simulink model "Testparentn"  (R2023b)
settings: Solver=FixedStepAuto  StartTime=0.0  StopTime=inf  RelTol=1e-3
undefined symbols (not defined in the file): lat, lon, Testparent2
libraries: androidcommunicationlib x3, androidaudiovideolib x2, androiduilib x2, visionsources x1
settings Model: Creator=Nihar  LastModifiedBy=kaver
settings OptimizationCC: EnhancedBackFolding=on  PassReuseOutputArgsAs=Individual arguments  ZeroExternalMemoryAtStartup=off  ZeroInternalMemoryAtStartup=off  MaxStackSize=64  OptimizeBlockOrder=speed  DifferentSizesBufferReuse=on  OptimizationCustomize=off  EfficientTunableParamExpr=on
settings DebuggingCC: ParameterTunabilityLossMsg=error
settings HardwareCC: ProdBitPerPointer=32  ProdBitPerSizeT=32  ProdBitPerPtrDiffT=32  ProdLargestAtomicInteger=Long  ProdLargestAtomicFloat=Double  ProdWordSize=32  ProdHWDeviceType=ARM Compatible->ARM Cortex
settings SFSimCC: MATLABDynamicMemAlloc=off
settings RTWCC: Description=Embedded Coder  SystemTargetFile=ert.tlc  HardwareBoard=Android Device  TLCOptions="-aInlineSetEventsForThisBaseRateFcn=TLC_FALSE -aSuppressMultiTaskScheduler=TLC_FALSE  -aRateBasedStepFcn=0"  TemplateMakefile=ert_default_tmf  RTWVerbose=off  Toolchain=Android SDK/NDK Tools
settings CodeAppCC: ForceParamTrailComments=on  IgnoreCustomStorageClasses=off  OperatorAnnotations=on  SimulinkDataObjDesc=on  SFDataObjDesc=on  InsertBlockDesc=on

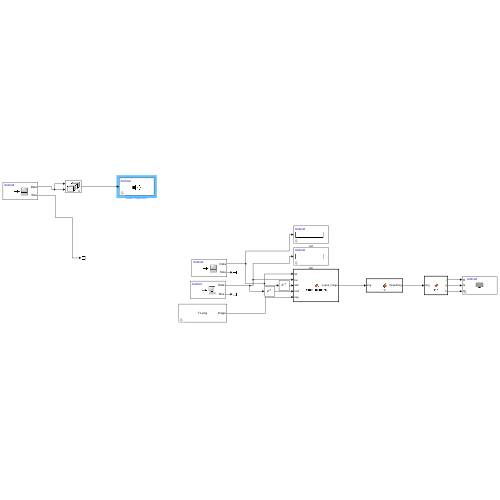
[thumbnail: Simulink's stored preview of the top-level diagram]
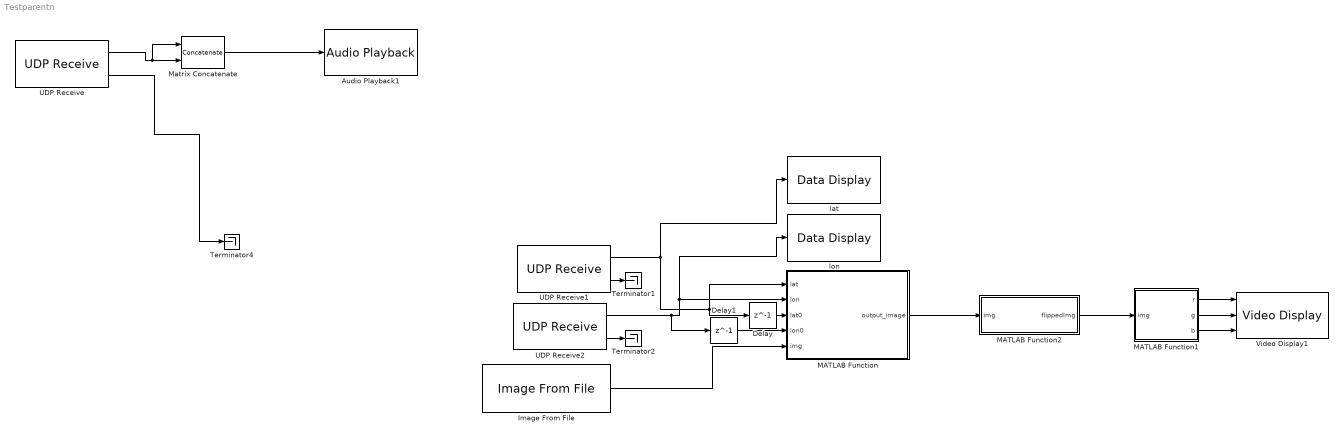
== system Testparentn ==
  Audio Playback1 : androidaudiovideolib/Audio Playback  SampleFreq=44100  AudioSamplingFreq=44100  SampleTime=0.1  DeviceStr=0  QueueDuration=0  BlockPlatform=Android
  Delay : Delay  DelayLength=1
  Delay1 : Delay  DelayLength=1
  Image From File : visionsources/Image From File  Tag=vipblks_nd  FileName=C:\Users\kaver\Downloads\TL.png  Ts=inf  imagePorts=One multidimensional signal  OutPortLabels=R|G|B  ImageDataType=uint8  sdImageDataType=uint(8)  Signed=on  WordLength=16  FractionLengthMode=User-defined  FractionLength=15
  MATLAB Function : MATLAB Function  TreatAsAtomicUnit=on
  MATLAB Function1 : MATLAB Function  TreatAsAtomicUnit=on
  MATLAB Function2 : MATLAB Function  TreatAsAtomicUnit=on
  Matrix Concatenate : Concatenate  Mode=Multidimensional array  ConcatenateDimension=2
  Terminator1 : Terminator
  Terminator2 : Terminator
  Terminator4 : Terminator
  UDP Receive : androidcommunicationlib/UDP Receive  localURL='0.0.0.0'  localPort=20000  remoteURL='0.0.0.0'  remotePort=-1  recvBufferSize=8192  signalDatatype=int16  dims=441  isVarSize=off  showBlockingTime=off  blockingTime=0  sampletime=0.01  blockPlatform=Android
  UDP Receive1 : androidcommunicationlib/UDP Receive  localURL='0.0.0.0'  localPort=35000  remoteURL='0.0.0.0'  remotePort=-1  recvBufferSize=8192  signalDatatype=double  dims=1  isVarSize=off  showBlockingTime=off  blockingTime=0  sampletime=0.01  blockPlatform=Android
  UDP Receive2 : androidcommunicationlib/UDP Receive  localURL='0.0.0.0'  localPort=25000  remoteURL='0.0.0.0'  remotePort=-1  recvBufferSize=8192  signalDatatype=double  dims=1  isVarSize=off  showBlockingTime=off  blockingTime=0  sampletime=0.01  blockPlatform=Android
  Video Display1 : androidaudiovideolib/Video Display  BlockPlatform=Android
  lat : androiduilib/Data Display  DataDisplayId=Testparent2/lat  Format=Float  Precision=6  SimulateUsing=Code generation  blockPlatform=Android
  lon : androiduilib/Data Display  DataDisplayId=Testparent2/lon  Format=Float  Precision=6  SimulateUsing=Code generation  blockPlatform=Android
  wires:
  Matrix Concatenate/1 -> Audio Playback1/1
  MATLAB Function/1(output_image) -> MATLAB Function2/1(img)
  UDP Receive2/2 -> Terminator2/1
  Delay/1 -> MATLAB Function/3(lat0)
  UDP Receive1/2 -> Terminator1/1
  Delay1/1 -> MATLAB Function/4(lon0)
  MATLAB Function1/1(r) -> Video Display1/1
  MATLAB Function1/3(b) -> Video Display1/3
  MATLAB Function1/2(g) -> Video Display1/2
  MATLAB Function2/1(flippedImg) -> MATLAB Function1/1(img)
  UDP Receive2/1 -> Delay1/1, lon/1, MATLAB Function/2(lon)
  Image From File/1 -> MATLAB Function/5(img)
  UDP Receive1/1 -> lat/1, MATLAB Function/1(lat), Delay/1
  UDP Receive/2 -> Terminator4/1
  UDP Receive/1 -> Matrix Concatenate/1, Matrix Concatenate/2

== matlab function Testparentn/MATLAB Function1 ==
  data: img input; r output; g output; b output
function [r,g,b] = fcn(img)
    r = img(:,:,1);
    g = img(:,:,2);
    b = img(:,:,3);
end

== matlab function Testparentn/MATLAB Function ==
  data: lat input; lon input; lat0 input; lon0 input; output_image output; img input
function output_image  = image_mapping(lat,lon,lat0,lon0,img)
    map_width = 883;
    map_height = 675;
    if(lat == 0)
        lat = lat0;
    end
    if(lon == 0)
        lon = lon0;
    end
    X = [83, 620, 640, 80, 441];
    Lx = [23.211144, 23.211170, 23.209616, 23.209530, 23.209997];
    Y = [70, 61, 427, 444, 337];
    Ly = [72.6833273, 72.685835, 72.685929, 72.683318, 72.685008];
    
    yL = zeros(map_height, 1);
    xL = zeros(1,map_width);

    for y = 1:map_height
            w_Y = ((y - Y(2)) * (y - Y(3)) * (y - Y(4)) * (y - Y(5))) / ((Y(1) - Y(2)) * (Y(1) - Y(3)) * (Y(1) - Y(4)) * (Y(1) - Y(5)));
            w_Y1 = ((y - Y(1)) * (y - Y(3)) * (y - Y(4)) * (y - Y(5))) / ((Y(2) - Y(1)) * (Y(2) - Y(3)) * (Y(2) - Y(4)) * (Y(2) - Y(5)));
            w_Y2 = ((y - Y(1)) * (y - Y(2)) * (y - Y(4)) * (y - Y(5))) / ((Y(3) - Y(1)) * (Y(3) - Y(2)) * (Y(3) - Y(4)) * (Y(3) - Y(5)));
            w_Y3 = ((y - Y(1)) * (y - Y(2)) * (y - Y(3)) * (y - Y(5))) / ((Y(4) - Y(1)) * (Y(4) - Y(2)) * (Y(4) - Y(3)) * (Y(4) - Y(5)));
            w_Y4 = ((y - Y(1)) * (y - Y(2)) * (y - Y(3)) * (y - Y(4))) / ((Y(5) - Y(1)) * (Y(5) - Y(2)) * (Y(5) - Y(3)) * (Y(5) - Y(4)));
            yL(y) = (w_Y * Lx(1)) + (w_Y1 * Lx(2)) + (w_Y2 * Lx(3)) + (w_Y3 * Lx(4)) + (w_Y4 * Lx(5));

    end
    for x = 1:map_width
            w_X = ((x - X(2)) * (x - X(3)) * (x - X(4)) * (x - X(5))) / ((X(1) - X(2)) * (X(1) - X(3)) * (X(1) - X(4)) * (X(1) - X(5)));
            w_X1 = ((x - X(1)) * (x - X(3)) * (x - X(4)) * (x - X(5))) / ((X(2) - X(1)) * (X(2) - X(3)) * (X(2) - X(4)) * (X(2) - X(5)));
            w_X2 = ((x - X(1)) * (x - X(2)) * (x - X(4)) * (x - X(5))) / ((X(3) - X(1)) * (X(3) - X(2)) * (X(3) - X(4)) * (X(3) - X(5)));
            w_X3 = ((x - X(1)) * (x - X(2)) * (x - X(3)) * (x - X(5))) / ((X(4) - X(1)) * (X(4) - X(2)) * (X(4) - X(3)) * (X(4) - X(5)));
            w_X4 = ((x - X(1)) * (x - X(2)) * (x - X(3)) * (x - X(4))) / ((X(5) - X(1)) * (X(5) - X(2)) * (X(5) - X(3)) * (X(5) - X(4)));
            xL(x) = (w_X * Ly(1)) + (w_X1 * Ly(2)) + (w_X2 * Ly(3)) + (w_X3 * Ly(4)) + (w_X4 * Ly(5));
     end
    
   
    
   
    [~, idx_y] = min(abs(yL - lat));
    [~, idx_x] = min(abs(xL - lon));
    min(abs(xL-lon))
    Xi = idx_x;
   
    Yi = idx_y;
    
    output_image = img;
    circle_radius = 7;
    % Ensure the circle coordinates are within bounds
    
    x = max(min(round(Xi), map_width), 1);
    y = max(min(round(Yi), map_height), 1);
    

    % Draw the filled circle manually
    for i = max(1, y - circle_radius):min(map_height, y + circle_radius)
        for j = max(1, x - circle_radius):min(map_width, x + circle_radius)
            if ((i - y)^2 + (j - x)^2) <= circle_radius^2
                output_image(i, j, 1) = 0; % Red channel
                output_image(i, j, 2) = 233;   % Green channel
                output_image(i, j, 3) = 226;   % Blue channel
            end
        end
    end
end

== matlab function Testparentn/MATLAB Function2 ==
  data: img input; flippedImg output
function flippedImg = flip(img)
    flippedImg = img(:, end:-1:1, :);
end
